simulink model "test_sim2"  (R2022b)
settings: Solver=ode4  StartTime=0.0  StopTime=50.0  FixedStep=0.01  RelTol=1e-3
values from neighbouring files (symbols this model uses):
  tau1 = 0.5    [paraset.m]
settings Model: Creator=user  LastModifiedBy=user
settings DataIOCC: ReturnWorkspaceOutputs=off

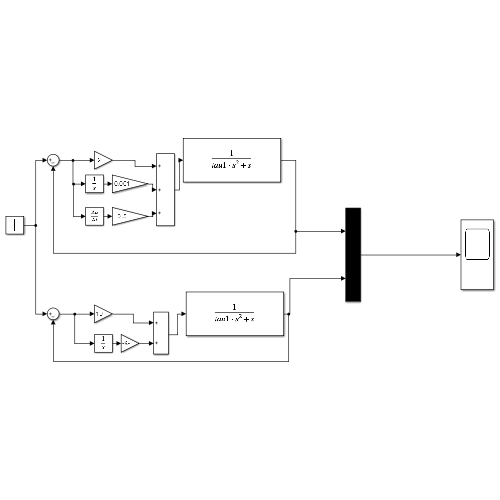
[thumbnail: Simulink's stored preview of the top-level diagram]
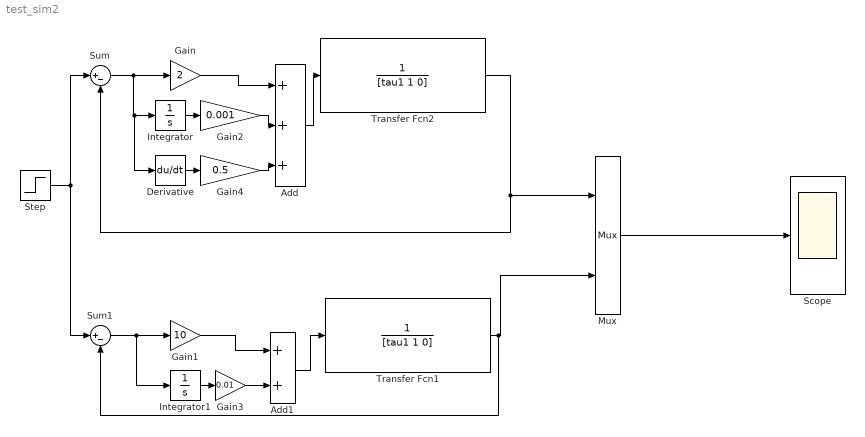
== system test_sim2 ==
  Add : Sum  Inputs=+++
  Add1 : Sum
  Derivative : Derivative
  Gain : Gain  Gain=2
  Gain1 : Gain  Gain=10
  Gain2 : Gain  Gain=0.001
  Gain3 : Gain  Gain=0.01
  Gain4 : Gain  Gain=0.5
  Integrator : Integrator
  Integrator1 : Integrator
  Mux : Mux  Inputs=2
  Scope : Scope
  Step : Step  After=100  SampleTime=0
  Sum : Sum  Inputs=|+-
  Sum1 : Sum  Inputs=|+-
  Transfer Fcn1 : TransferFcn  Denominator=[tau1 1 0]
  Transfer Fcn2 : TransferFcn  Denominator=[tau1 1 0]
  wires:
  Transfer Fcn2/1 -> Sum/2, Mux/1
  Transfer Fcn1/1 -> Mux/2, Sum1/2
  Mux/1 -> Scope/1
  Sum/1 -> Derivative/1, Integrator/1, Gain/1
  Step/1 -> Sum1/1, Sum/1
  Sum1/1 -> Integrator1/1, Gain1/1
  Integrator/1 -> Gain2/1
  Integrator1/1 -> Gain3/1
  Gain2/1 -> Add/2
  Gain/1 -> Add/1
  Add/1 -> Transfer Fcn2/1
  Gain3/1 -> Add1/2
  Gain1/1 -> Add1/1
  Add1/1 -> Transfer Fcn1/1
  Gain4/1 -> Add/3
  Derivative/1 -> Gain4/1
